simulink model "pidmodel_org"  (Simulink 10.0)
settings: Solver=ode45  StartTime=0.0  StopTime=10  RelTol=1e-3  EnableMultiTasking=on
InitFcn:
  | param
undefined symbols (not defined in the file): AP, can_ctrl
libraries: cstblocks x1
settings Model: Creator=paul  LastModifiedBy=bhisma
settings DataIOCC: LimitDataPoints=on
settings DebuggingCC: SolverPrmCheckMsg=warning
settings GRTTargetCC: GeneratePreprocessorConditionals=Disable all  CombineOutputUpdateFcns=on  GRTInterface=off
settings ConfigComp: CovExternalEMLEnable=off

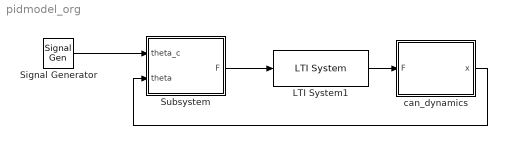
== system pidmodel_org ==
  LTI System1 : cstblocks/LTI System  sys=C  IC=[]
  Signal Generator : SignalGenerator  WaveForm=square  Amplitude=pi/3
  Subsystem : Subsystem
  can_dynamics : Subsystem
  wires:
  Signal Generator/1 -> Subsystem/1(theta_c)
  can_dynamics/1(x) -> Subsystem/2(theta)
  LTI System1/1 -> can_dynamics/1(F)
  Subsystem/1(F) -> LTI System1/1

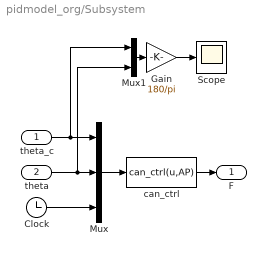
== system pidmodel_org/Subsystem ==
  theta_c : Inport
  theta : Inport  Port=2
  Clock : Clock
  Gain : Gain  Gain=180/pi
  Mux : Mux  Inputs=3
  Mux1 : Mux  Inputs=2
  Scope : Scope
  can_ctrl : MATLABFcn  MATLABFcn=can_ctrl(u,AP)  OutputDimensions=1  SampleTime=AP.Ts
  F : Outport
  wires:
  theta_c/1 -> Mux1/1, Mux/1
  Mux/1 -> can_ctrl/1
  Gain/1 -> Scope/1
  Mux1/1 -> Gain/1
  can_ctrl/1 -> F/1
  Clock/1 -> Mux/3
  theta/1 -> Mux1/2, Mux/2

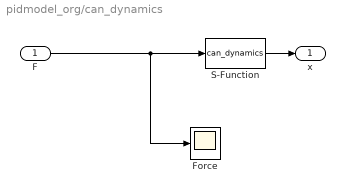
== system pidmodel_org/can_dynamics ==
  F : Inport
  Force : Scope
  S-Function : S-Function  FunctionName=can_dynamics  Parameters=AP  SFunctionDeploymentMode=off  EnableBusSupport=off
  x : Outport
  wires:
  F/1 -> Force/1, S-Function/1
  S-Function/1 -> x/1
